simulink model "SARSA_ET_block_simulink"  (R2022a)
settings: Solver=VariableStepAuto  StartTime=0.0  StopTime=10.0  RelTol=1e-3
values from neighbouring files (symbols this model uses):
  A = 3*3    (= 9)    [Configuration.m]    (also in test_sim.mat; test_sim_10000Ep_v10.mat; test_sim_10000Ep_v12_G_oldScen.mat; test_sim_10000Ep_v1_dist.mat)
  alpha = 1e-3    (= 0.001)    [Configuration.m]
  d = A*N*nCells    (= 699840)    [Configuration.m]    (also in get_features.m = A*N*nCells; test_sim.mat = 18432; test_sim_10000Ep_v10.mat; test_sim_10000Ep_v12_G_oldScen.mat)
  epsilon = 1e-1    (= 0.1)    [Configuration.m]
  gamma = 0.9    [Configuration.m]
  gridvx = zeros(N, length(TVX))    [construct_tiles.m]    (also in test_sim.mat = [-3.33333333333 -3.21428571429 -3.09523809524 -2.97619047619; test_sim_10000Ep_v10.mat = [-2.8 -2.75555555556 -2.71111111111 -2.66666666667 -2.622222; test_sim_10000Ep_v12_G_oldScen.mat = [-2.8 -2.75555555556 -2.71111111111 -2.66666666667 -2.622222; test_sim_10000Ep_v1_dist.mat = [-2.8 -2.75555555556 -2.71111111111 -2.66666666667 -2.622222)
  gridvy = zeros(N, length(TVY))    [construct_tiles.m]    (also in test_sim.mat = [-3.33333333333 -3.16666666667 -3 -2.83333333333 -2.66666666; test_sim_10000Ep_v10.mat = [-28 -27.3777777778 -26.7555555556 -26.1333333333 -25.511111; test_sim_10000Ep_v12_G_oldScen.mat = [-28 -27.3777777778 -26.7555555556 -26.1333333333 -25.511111; test_sim_10000Ep_v1_dist.mat = [-28 -27.3777777778 -26.7555555556 -26.1333333333 -25.511111)
  gridx = zeros(N, length(TX))    [construct_tiles.m]    (also in test_sim.mat = [-8.33333333333 -8.18452380952 -8.03571428571 -7.8869047619 ; test_sim_10000Ep_v10.mat = [-5 -4.94444444444 -4.88888888889 -4.83333333333 -4.77777777; test_sim_10000Ep_v12_G_oldScen.mat = [-5 -4.94444444444 -4.88888888889 -4.83333333333 -4.77777777; test_sim_10000Ep_v1_dist.mat = [-5 -4.94444444444 -4.88888888889 -4.83333333333 -4.77777777)
  gridy = zeros(N, length(TY))    [construct_tiles.m]    (also in test_sim.mat = [-16.6666666667 -16.3095238095 -15.9523809524 -15.5952380952; test_sim_10000Ep_v10.mat = [-2 -1.93333333333 -1.86666666667 -1.8 -1.73333333333 -1.666; test_sim_10000Ep_v12_G_oldScen.mat = [-2 -1.93333333333 -1.86666666667 -1.8 -1.73333333333 -1.666; test_sim_10000Ep_v1_dist.mat = [0.4 0.453333333333 0.506666666667 0.56 0.613333333333 0.666)
  gridyaw = [-504 -489.6 -475.2 -460.8 -446.4 -432 -417.6 -403.2 -388.8 -374.4 -360 -345.6 ... (70 elements, 10x7)]    [test_sim_10000Ep_v10.mat]    (also in test_sim_10000Ep_v12_G_oldScen.mat; test_sim_10000Ep_v1_dist.mat = [-126 -122.4 -118.8 -115.2 -111.6 -108 -104.4 -100.8 -97.2 -; test_sim_1000Ep.mat = [-600 -570 -540 -510 -480 -450 -420 -390 -360 -330 -300 -270; test_sim_1000Ep_v2newparam.mat = [-600 -570 -540 -510 -480 -450 -420 -390 -360 -330 -300 -270)
  lambda = 1    [Configuration.m]
  M = 5    [Configuration.m]    (also in test_sim.mat = 3; test_sim_10000Ep_v10.mat; test_sim_10000Ep_v12_G_oldScen.mat; test_sim_10000Ep_v1_dist.mat)
  N = 10    [Configuration.m]    (also in test_sim.mat = 8; test_sim_10000Ep_v10.mat; test_sim_10000Ep_v12_G_oldScen.mat; test_sim_10000Ep_v1_dist.mat)
settings Model: Creator=User  LastModifiedBy=User

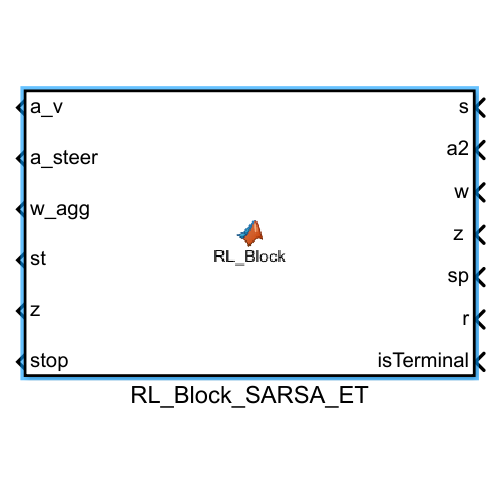
[thumbnail: Simulink's stored preview of the top-level diagram]
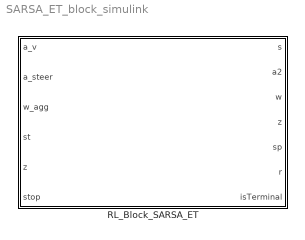
== system SARSA_ET_block_simulink ==
  RL_Block_SARSA_ET : MATLAB Function  TreatAsAtomicUnit=on

== matlab function SARSA_ET_block_simulink/RL_Block_SARSA_ET ==
  settings: updateMethod=DISCRETE  sampleTime=Ts
  data: a_v output [..200]; s input; a2 input; w input; z input; a_steer output; sp input; r input; isTerminal input; w_agg output; st output; z output; stop output; gridx parameter; gridy parameter; gridvx parameter; gridvy parameter; M parameter; N parameter; epsilon parameter; gamma parameter; alpha parameter; A parameter; d parameter; gridyaw parameter; lambda parameter
function [a_v, a_steer, w_agg, st, z, stop] = RL_Block(s, a2, w, z, sp, r, isTerminal, gridx, gridy, gridvx, gridvy, M, N, epsilon, gamma, alpha, A, d, gridyaw, lambda)

coder.extrinsic('assignin') % altrimenti devo usare toWorkspace

% a = [a1;a2] vect colonna con [(1/2/3);(1/2/3)] 
% come gestisco agg parametri w

%steps = steps + 1; % così mostriamo num passi

stop = 0;

% mi serve stato attuale e stato successivo
% creare consistenza tra stato precedente e successivo
a = sub2ind([3 3], a2(1), a2(2));
ae = a;
x = get_features(s, a, gridx, gridy, gridvx, gridvy, gridyaw, M, N, A, d); % features stato attuale
%[sp, r,isTerminal] = dynamics_mountain_car(s, a, lbx, ubx, lbv, ubv); % questo lo prendo da input da modello simulink
if isTerminal
    delta = r - w'*x;
    %assignin("base", "w", w_agg)
    stop = 1;
else                        % da epsilon li devo passare come parameti
    ap = eps_greedy(sp, w, epsilon, gridx, gridy, gridvx, gridvy, gridyaw, M, N, A, d); % azione success
    xp = get_features(sp, ap, gridx, gridy, gridvx, gridvy, gridyaw, M, N, A, d); % features stato success
    delta = r + gamma*w'*xp - w'*x;
    ae = ap;
end
z = gamma*lambda*z + x;
w_agg = w + alpha*delta*z;

if isTerminal
    assignin("base", "w", w_agg)
end
st = sp; % aggiorno              mi manca riferimento ad azione precedente caso isTerminal
%a_v = 0;
[b1,b2] = ind2sub([3 3],ae);

% [1 2 3] vanno mappati su -1,0, con (-2)

if(b1 == 1)
    a_v = 1;
elseif(b1 == 2)
    a_v = 2;
else
    a_v = 3;
end

if(b2 == 1)
    a_steer = 1;
elseif(b2 == 2)
    a_steer = 2;
else
    a_steer = 3;
end

%[a_v,a_steer] = ind2sub([3 3],ae);
%a_v = ones(1,1);
%a_v = b1;
%a_steer = b2;
% cos' mi dava errore di dimensione variabile

%assignin("base", "az_1", b1);

end



%%%%%%%%%%%%%%%%%%%%%%%%%%%%%%%%%%%%%%%%%%%%%%%%%%
%              FUNZIONI AUSILIARE
%%%%%%%%%%%%%%%%%%%%%%%%%%%%%%%%%%%%%%%%%%%%%%%%%%

% Funzione che mi restituisce l'azione epsgreedy da scegliere

function a = eps_greedy(s, w, eps, gridx, gridy, gridvx, gridvy, gridyaw, M, N, A, d)

if rand < eps   % azione random
    a = randi(A); % da 1 a 9 se uso indice
else
    q = zeros(A, 1);
    for a = 1:A  % valuto tutte le azioni che posso prendere
        q(a) = w'*get_features(s, a, gridx, gridy, gridvx, gridvy, gridyaw, M, N, A, d); % approsimazione della funz qualità
    end        % pesi per vett features
    a = find(q == max(q), 1, 'first'); % scelgo quella con funz qualità massima
end
end


function x = get_features(s, a, gridx, gridy, gridvx, gridvy, gridyaw, M, N, A, d)

%coder.extrinsic('assignin')

% numero celle, +1 perchè ne ho aggiunta una
%nCells = (M + 1)^4; % dimensione features per una cella
%d = A*N*nCells; % dimensione vettore pesi da aggiornare
x = zeros(d, 1);
% va modificaro sta dimension var
for ii = 1 : N
    xxx = gridx(ii, :);
    yyy = gridy(ii, :);
    vxvxvx = gridvx(ii, :);
    vyvyvy = gridvy(ii, :);
    yawyawyaw = gridyaw(ii, :);
    % capire in quale cella mi trovo, trovo indice lungo x e lungo y
    ix = find(s(1) >= xxx(1:end-1) & s(1) <= xxx(2:end), 1, 'first');
    iy = find(s(2) >= yyy(1:end-1) & s(2) <= yyy(2:end), 1, 'first');
    ivx = find(s(3) >= vxvxvx(1:end-1) & s(3) <= vxvxvx(2:end), 1, 'first');
    ivy = find(s(4) >= vyvyvy(1:end-1) & s(4) <= vyvyvy(2:end), 1, 'first');
    iyaw = find(s(5) >= yawyawyaw(1:end-1) & s(5) <= yawyawyaw(2:end), 1, 'first');

    % a_ind = sub2ind([3 3],a(1),a(2)); non serve gli passo indice poi da
    % indice a azione quando la uso in dinamica
    % dato doppia dim dell'azione devo subind anche a ???

    % debug
    %pippo = struct('ix',{ix},'iy', {iy},'ivx', {ivx},'ivy', {ivy},'ii', {ii},'a', {a},'s', {s});
    %assignin("base","pippo",pippo);
    ind = sub2ind([M + 1, M + 1, M + 1, M + 1, M + 1, N, A], ix, iy, ivx, ivy, iyaw, ii, a);

    x(ind) = 1; % valore corrispondente alla cella
    % vett features ha un 1 per ogni griglia
end
end
